simulink model "lab_2"  (R2024a)
settings: Solver=VariableStepAuto  StartTime=0.0  StopTime=10.0  RelTol=1e-3
settings Model: Creator=lw53894  LastModifiedBy=lw53894

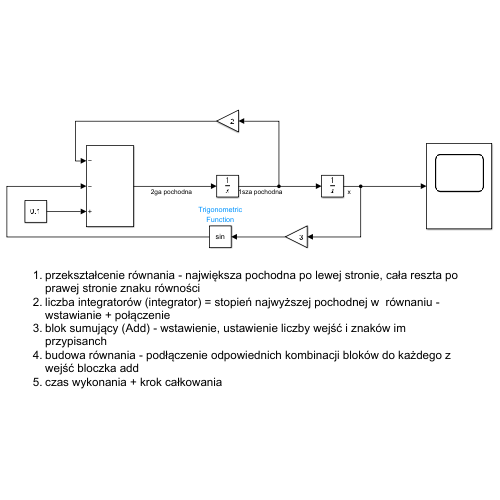
[thumbnail: Simulink's stored preview of the top-level diagram]
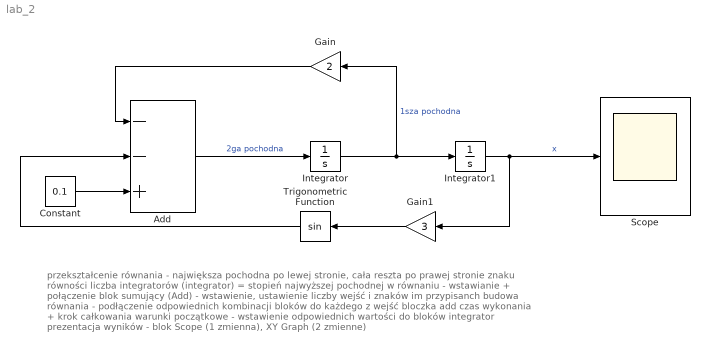
== system lab_2 ==
  note: przekształcenie równania - największa pochodna po lewej stronie, cała reszta po prawej stronie znaku równości
      | liczba integratorów (integrator) = stopień najwyższej pochodnej w równaniu - wstawianie + połączenie
      | blok sumujący (Add) - wstawienie, ustawienie liczby wejść i znaków im przypisanch
      | budowa równania - podłączenie odpowiednich kombinacji bloków do każdego z wejść bloczka add
      | czas wykonania + krok całkowania
      | warunki początkowe - wstawienie odpowiednich wartości do bloków integrator
      | prezentacja wyników - blok Scope (1 zmienna), XY Graph (2 zmienne)
  Add : Sum  Inputs=--+
  Constant : Constant  Value=0.1
  Gain : Gain  Gain=2
  Gain1 : Gain  Gain=3
  Integrator : Integrator  InitialCondition=2
  Integrator1 : Integrator
  Scope : Scope
  Trigonometric Function : Trigonometry
  wires:
  Integrator/1 -> Gain/1, Integrator1/1  "1sza pochodna"
  Add/1 -> Integrator/1  "2ga pochodna"
  Constant/1 -> Add/3
  Gain/1 -> Add/1
  Integrator1/1 -> Gain1/1, Scope/1  "x"
  Gain1/1 -> Trigonometric Function/1
  Trigonometric Function/1 -> Add/2
